simulink model "Model"  (R2015b)
settings: Solver=ode45  StartTime=0.0  StopTime=100  MaxStep=1e-3  RelTol=1e-3
undefined symbols (not defined in the file): K1, Kp, tau
settings Model: Creator=s3blanch  LastModifiedBy=s3blanch

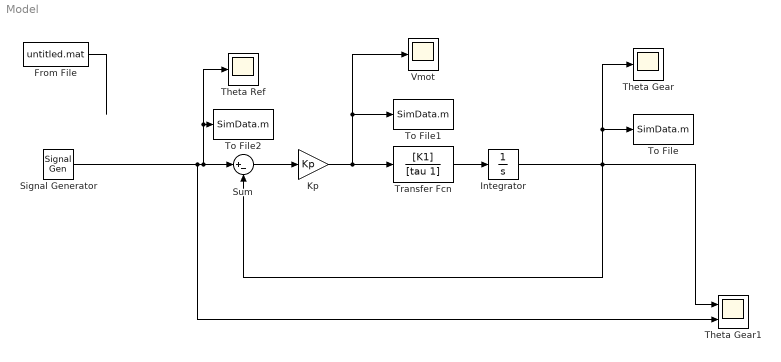
== system Model ==
  From File : FromFile  SampleTime=0
  Integrator : Integrator
  Kp : Gain  Gain=Kp
  Signal Generator : SignalGenerator  WaveForm=square  Amplitude=0.6  Frequency=0.05
  Sum : Sum  Inputs=|+-
  Theta Gear : Scope
  Theta Gear1 : Scope  NumInputPorts=2
  Theta Ref : Scope
  To File : ToFile  Filename=SimData.m  MatrixName=Og_sim
  To File1 : ToFile  Filename=SimData.m  MatrixName=Vmot_sim
  To File2 : ToFile  Filename=SimData.m  MatrixName=Oref_sim
  Transfer Fcn : TransferFcn  Numerator=[K1]  Denominator=[tau 1]
  Vmot : Scope
  wires:
  Signal Generator/1 -> Theta Gear1/2, To File2/1, Theta Ref/1, Sum/1
  Transfer Fcn/1 -> Integrator/1
  Kp/1 -> To File1/1, Vmot/1, Transfer Fcn/1
  Sum/1 -> Kp/1
  Integrator/1 -> Theta Gear1/1, Sum/2, To File/1, Theta Gear/1
  From File/1 -> ?
